simulink subsystem "Sustainer_Aerodynamics_old"  (R2023b)
settings: Solver=VariableStepAuto  StartTime=0.0  StopTime=10.0  RelTol=1e-3
undefined symbols (not defined in the file): ALPHA_axis3, ALT_axis1, CA_sustainer, CAQ_sustainer, CLL_sustainer, CLN_sustainer, CLP_sustainer, CLR_sustainer, CM_sustainer, CMAD_sustainer, CMQ_sustainer, CN_sustainer, CNAD_sustainer, CNP_sustainer, CNQ_sustainer, CNR_sustainer, CY_sustainer, CYP_sustainer, CYR_sustainer, F, Light, LREF, MIL, PHI_axis2, SREF, XCG_dry, XCP_sustainer
libraries: aerolibconvert2 x5, aerolibasang x2, simulink_extras x2, aerolibadyn x1, aerolibatmos2 x1, aerolibwind2 x1
settings Model: Creator=Andrew Radulovich  LastModifiedBy=thatf
settings ModelReferenceCC: EnableRefExpFcnMdlSchedulingChecks=on

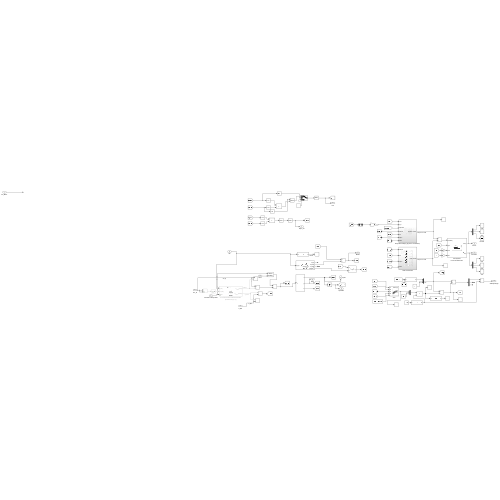
[thumbnail: Simulink's stored preview of the top-level diagram]
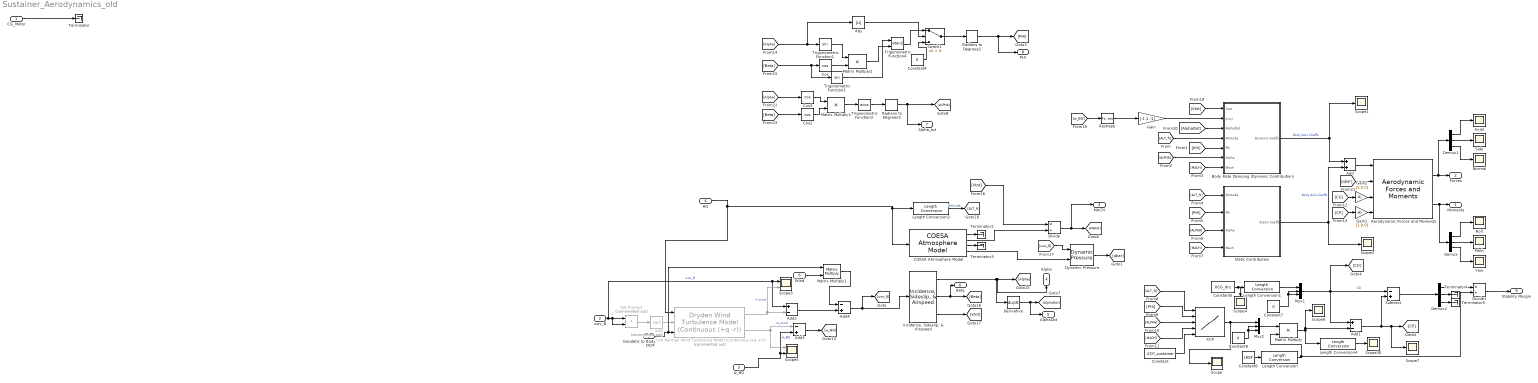
== system Sustainer_Aerodynamics_old ==
  CG_Motor : Inport
  uwv_B : Inport  Port=2
  w_BG : Inport  Port=3
  HG : Inport  Port=4
  Geodetic to Body DCM : Inport  Port=5
  Wind : Inport  Port=6
  Abs : Abs  SaturateOnIntegerOverflow=off
  Add : Sum
  Add1 : Sum  Inputs=+-
  Add2 : Sum  Inputs=+-
  Add3 : Sum  Inputs=-+
  Add4 : Sum  Inputs=-+
  "Aerodynamic Forces and Moments " : aerolibadyn/Aerodynamic Forces and Moments   inputAxes=Body  outputForceAxes=Body  outputMomentAxes=Body  S=SREF*0.0254*0.0254  b=LREF*0.0254  cbar=LREF*0.0254
  Axial : Scope
  "Body Rate Damping (Dynamic Contribution) " : Subsystem
  COESA Atmosphere Model : aerolibatmos2/COESA Atmosphere Model  units=Metric (MKS)  spec=1976 COESA-extended U.S. Standard Atmosphere  model=Profile  profile_var=High temperature  profile_percent=1%  profile_alt=5 km (16404 ft)  envelope_var=High temperature  envelope_percent=1%  action=None
  Constant : Constant  Value=XCP_sustainer  VectorParams1D=off
  Constant4 : Constant  Value=0
  Constant5 : Constant  Value=XCG_dry
  Constant6 : Constant  Value=LREF
  Constant7 : Constant  Value=0
  Constant8 : Constant  Value=0
  Cos : Trigonometry  Operator=cos
  Cos2 : Trigonometry  Operator=cos
  Cos3 : Trigonometry  Operator=cos
  Demux : Demux  Outputs=3
  Demux1 : Demux  Outputs=3
  Demux2 : Demux  Outputs=3
  Derivative : Derivative
  Divide : Product  Inputs=*/
  Divide1 : Product  Inputs=*/
  Dot Product : DotProduct  Commented=on  OutDataTypeStr=Inherit: Inherit via internal rule
  Dynamic Pressure : aerolibasang/Dynamic Pressure
  Gain : Gain  Gain=[-1,1,-1]
  Gain1 : Gain  Gain=[1,0,0]
  Gain2 : Gain  Gain=[1,0,0]
  "Incidence, Sideslip, & Airspeed" : aerolibasang/Incidence, Sideslip, & Airspeed
  Length Conversion : aerolibconvert2/Length Conversion  IU=in  OU=m
  Length Conversion1 : aerolibconvert2/Length Conversion  IU=in  OU=m
  Length Conversion2 : aerolibconvert2/Length Conversion  IU=m  OU=ft
  Length Conversion4 : aerolibconvert2/Length Conversion  IU=m  OU=in
  Matrix Multiply : Product
  Matrix Multiply1 : Product  Multiplication=Matrix(*)
  Matrix Multiply2 : Product
  Matrix Multiply3 : Product
  Mux1 : Mux  Inputs=3
  Mux2 : Mux  Inputs=3
  Normal : Scope
  Pitch : Scope
  Radians to Degrees2 : simulink_extras/Transformations/Radians to Degrees
  Radians to Degrees3 : simulink_extras/Transformations/Radians to Degrees
  Reshape : Reshape  OutputDimensionality=Row vector (2-D)
  Roll : Scope
  Scope{,1..2,4,6..7,30} (7 alike) : Scope
  Scope3 : Scope  NumInputPorts=2
  Scope5 : Scope  NumInputPorts=2
  Side : Scope
  Sqrt : Sqrt  Commented=on
  Static Contribution : Subsystem
  Subtract : Sum  Inputs=-+
  Switch1 : Switch  Criteria=u2 > Threshold  SaturateOnIntegerOverflow=off  InputSameDT=off
  Terminator{,2..5} (5 alike) : Terminator
  Trigonometric Function1 : Trigonometry
  Trigonometric Function2 : Trigonometry
  Trigonometric Function3 : Trigonometry  Operator=acos
  Trigonometric Function4 : Trigonometry  Operator=atan2
  Von Karman Wind Turbulence Model (Continuous (+q +r)) : aerolibwind2/Dryden Wind Turbulence Model  (Continuous (+q -r))  Commented=on  units=Metric (MKS)  spec=MIL-F-8785C  model=Continuous Von Karman (+q +r)  W20=15  Wdeg=0  TurbProb=10^-2 - Light  L_high=762  Wingspan=10  ts=0.1  Seed=[23341 23342 23343 23344]  T_on=on
  XCP : Lookup_n-D  NumberOfTableDimensions=4  BreakpointsForDimension1=ALT_axis1  BreakpointsForDimension2=PHI_axis2  BreakpointsForDimension3=ALPHA_axis3  BreakpointsForDimension4=MACH_axis4  TableSource=Input port  Table=reshape(repmat([4 5 6;16 19 20;10 18 23],1,2),[3,3,2])  InternalRulePriority=Speed  RndMeth=Simplest
      settings: InputPortMap=u0,u1,u2,u3,p221
  Yaw : Scope
  Moments : Outport
  Forces : Outport  Port=2
  MACH : Outport  Port=3
  Alpha : Outport  Port=4
  AlphaDot : Outport  Port=5
  Beta : Outport  Port=6
  Alpha_tot : Outport  Port=7
  PHI : Outport  Port=8
  Stability Margin : Outport  Port=9
  wires:
  CG_Motor/1 -> Terminator/1
  [ALPHA] -> XCP/3
  Abs/1 -> Switch1/2
  XCP/1 -> Scope/1, Mux2/1
  Divide/1 -> [MACH], MACH/1
  [Alpha] -> Cos3/1
  Trigonometric Function4/1 -> Switch1/1
  Cos3/1 -> Matrix Multiply3/1
  [uwv_B] -> Dynamic Pressure/1
  "Incidence, Sideslip, & Airspeed"/2 -> [Beta], Beta/1
  Trigonometric Function2/1 -> Trigonometric Function4/1
  Dynamic Pressure/1 -> [qbar]
  Gain/1 -> "Body Rate Damping (Dynamic Contribution) "/2(p,q,r)
  Length Conversion2/1 -> [ALT_ft]  "Altitude"
  COESA Atmosphere Model/3 -> Terminator3/1
  Static Contribution/1(Static Coeffs) -> Scope2/1, Add/2  "Body Axis Coeffs"
  Length Conversion/1 -> Matrix Multiply/2, Divide1/2
  Switch1/1 -> Radians to Degrees2/1
  [PHI] -> Static Contribution/2(Phi)
  [CP] -> Gain1/1
  Constant4/1 -> Switch1/3
  Gain1/1 -> "Aerodynamic Forces and Moments "/4
  Demux1/2 -> Side/1
  Constant6/1 -> Length Conversion/1
  [CG] -> Gain2/1
  Radians to Degrees2/1 -> [PHI], PHI/1
  Demux1/1 -> Axial/1
  [MACH] -> XCP/4
  Mux2/1 -> Matrix Multiply/1
  Add1/1 -> [CP], Scope7/1, Subtract/2
  "Aerodynamic Forces and Moments "/2 -> Demux/1, Moments/1
  Matrix Multiply/1 -> Length Conversion4/1, Add1/2, Scope6/1
  [MACH] -> Static Contribution/4(Mach)
  [PHI] -> XCP/2
  Gain2/1 -> "Aerodynamic Forces and Moments "/3
  "Incidence, Sideslip, & Airspeed"/1 -> Derivative/1, [Alpha], Alpha/1
  [AlphaDot] -> "Body Rate Damping (Dynamic Contribution) "/3(AlphaDot)
  Length Conversion1/1 -> Mux1/1
  Demux/3 -> Yaw/1
  Demux1/3 -> Normal/1
  [Vtot] -> "Body Rate Damping (Dynamic Contribution) "/1(Vtot)
  "Body Rate Damping (Dynamic Contribution) "/1("Dynamic Coeffs ") -> Add/1, Scope1/1  "Body Axis Coeffs"
  [ALT_ft] -> "Body Rate Damping (Dynamic Contribution) "/4(Altitude)
  Constant/1 -> XCP/5
  [Beta] -> Trigonometric Function2/1, Cos/1
  [qbar] -> "Aerodynamic Forces and Moments "/2
  Add/1 -> "Aerodynamic Forces and Moments "/1
  [ALT_ft] -> XCP/1
  Length Conversion4/1 -> Scope30/1
  Matrix Multiply3/1 -> Trigonometric Function3/1
  Cos/1 -> Matrix Multiply2/2
  Derivative/1 -> [AlphaDot], AlphaDot/1
  HG/1 -> Length Conversion2/1, COESA Atmosphere Model/1, Von Karman Wind Turbulence Model (Continuous (+q +r))/1
  Constant7/1 -> Mux1/2, Mux1/3
  Dot Product/1 -> Sqrt/1
  Cos2/1 -> Matrix Multiply3/2
  COESA Atmosphere Model/2 -> Divide/2
  [MACH] -> "Body Rate Damping (Dynamic Contribution) "/7(Mach)
  w_BG/1 -> Scope5/2, Add3/2  "w_BG"
  Trigonometric Function1/1 -> Matrix Multiply2/1
  Mux1/1 -> Add1/1, [CG], Subtract/1  "CG"
  Radians to Degrees3/1 -> [ALPHA], Alpha_tot/1
  Demux/1 -> Roll/1
  Trigonometric Function3/1 -> Radians to Degrees3/1
  Add2/1 -> Add4/2
  Matrix Multiply1/1 -> Add4/1
  Wind/1 -> Matrix Multiply1/2
  [PHI] -> "Body Rate Damping (Dynamic Contribution) "/5(Phi)
  "Incidence, Sideslip, & Airspeed"/3 -> [Vtot]
  COESA Atmosphere Model/4 -> Dynamic Pressure/2
  [ALPHA] -> "Body Rate Damping (Dynamic Contribution) "/6(Alpha)
  Add3/1 -> [w_BG]
  COESA Atmosphere Model/1 -> Terminator2/1
  Sqrt/1 -> Von Karman Wind Turbulence Model (Continuous (+q +r))/2
  Constant5/1 -> Length Conversion1/1, Scope4/1
  [Beta] -> Cos2/1
  Von Karman Wind Turbulence Model (Continuous (+q +r))/2 -> Scope5/1, Add3/1  "w_wind"
  [Vtot] -> Divide/1
  [ALPHA] -> Static Contribution/3(Alpha)
  Add4/1 -> [uwv_B], "Incidence, Sideslip, & Airspeed"/1
  Reshape/1 -> Gain/1
  Matrix Multiply2/1 -> Trigonometric Function4/2
  Geodetic to Body DCM/1 -> Von Karman Wind Turbulence Model (Continuous (+q +r))/3, Matrix Multiply1/1
  Demux/2 -> Pitch/1
  [w_BG] -> Reshape/1
  uwv_B/1 -> Dot Product/1, Dot Product/2, Scope3/1, Add2/1  "uwv_B"
  [Alpha] -> Trigonometric Function1/1, Abs/1
  [ALT_ft] -> Static Contribution/1(Altitude)
  Constant8/1 -> Mux2/2, Mux2/3
  "Aerodynamic Forces and Moments "/1 -> Forces/1, Demux1/1
  Von Karman Wind Turbulence Model (Continuous (+q +r))/1 -> Scope3/2, Add2/2  "V wind"
  Subtract/1 -> Demux2/1
  Demux2/1 -> Divide1/1
  Demux2/2 -> Terminator4/1
  Demux2/3 -> Terminator5/1
  Divide1/1 -> Stability Margin/1

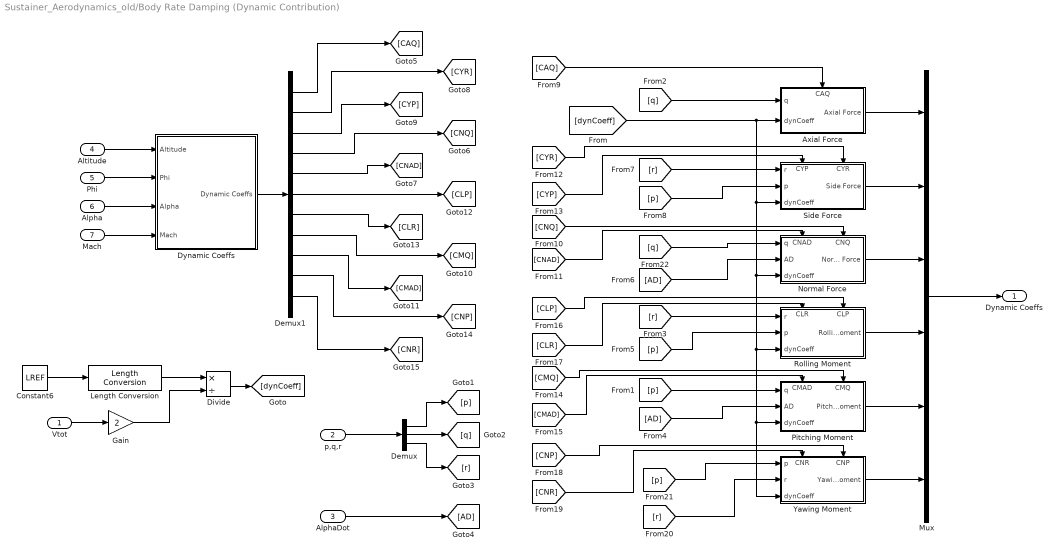
== system Sustainer_Aerodynamics_old/Body Rate Damping (Dynamic Contribution)  ==
  Vtot : Inport
  p,q,r : Inport  Port=2
  AlphaDot : Inport  Port=3
  Altitude : Inport  Port=4
  Phi : Inport  Port=5
  Alpha : Inport  Port=6
  Mach : Inport  Port=7
  Axial Force : Subsystem
      settings: PortSchema="{\"entries\":[{\"content\":{\"sides\":[{\"content\":{\"connectorIds\":[\"In1\",\"In2\"]},\"type\":\"ConnectorPlacement.EquallySpacedRectSide\",\"uuid\":\"567ace9e-aa72-447b-a995-1912c2144b72\"},{\"content\":{\"connectorIds\":[\"Out1\"],\"side\":\"RIGHT\"},\"type\":\"ConnectorPlacement.EquallySpacedRectSide\",\"uuid\":\"f61a370b-a555-422d-b0aa-b7ff6aed3edf\"},{\"content\":{\"connectorIds\":[\"In3\"],\"side\":\"TOP\"},\"type\":\"ConnectorPlacement.EquallySpacedRectSide\",\"uuid\":\"bbb221a2-e351-4e94-b4cf-9d8a77c477bc\"}]},\"type\":\"ConnectorPlacement.EquallySpacedConnector\",\"uuid\":\"32afc2d8-df0e-48c6-a674-90055023081f\"}],\"packageUris\":[\"http://schema.mathworks.com/mf0/Connector/R2020b\"],\"version\":\"1.0\"}"
  Constant6 : Constant  Value=LREF
  Demux : Demux  Outputs=3
  Demux1 : Demux  Outputs=11
  Divide : Product  Inputs=*/
  Dynamic Coeffs : Subsystem
  Gain : Gain  Gain=2
  Length Conversion : aerolibconvert2/Length Conversion  IU=in  OU=m
  Mux : Mux  Inputs=6
  Normal Force : Subsystem
      settings: PortSchema="{\"entries\":[{\"content\":{\"sides\":[{\"content\":{\"connectorIds\":[\"In1\",\"In2\",\"In3\"]},\"type\":\"ConnectorPlacement.EquallySpacedRectSide\",\"uuid\":\"36c1ca9e-f728-46fa-a5e1-3a4eef93369b\"},{\"content\":{\"connectorIds\":[\"Out1\"],\"side\":\"RIGHT\"},\"type\":\"ConnectorPlacement.EquallySpacedRectSide\",\"uuid\":\"48421245-83fe-4d4e-9595-34bafe35022f\"},{\"content\":{\"connectorIds\":[\"In4\",\"In5\"],\"side\":\"TOP\"},\"type\":\"ConnectorPlacement.EquallySpacedRectSide\",\"uuid\":\"de332918-1e12-41a2-8ccc-a9221aaa9415\"}]},\"type\":\"ConnectorPlacement.EquallySpacedConnector\",\"uuid\":\"0485d59f-61a8-483f-be32-e9ca6bf2e6bf\"}],\"packageUris\":[\"http://schema.mathworks.com/mf0/Connector/R2020b\"],\"version\":\"1.0\"}"
  Pitching Moment : Subsystem
      settings: PortSchema="{\"entries\":[{\"content\":{\"sides\":[{\"content\":{\"connectorIds\":[\"In1\",\"In2\",\"In3\"]},\"type\":\"ConnectorPlacement.EquallySpacedRectSide\",\"uuid\":\"36c1ca9e-f728-46fa-a5e1-3a4eef93369b\"},{\"content\":{\"connectorIds\":[\"Out1\"],\"side\":\"RIGHT\"},\"type\":\"ConnectorPlacement.EquallySpacedRectSide\",\"uuid\":\"48421245-83fe-4d4e-9595-34bafe35022f\"},{\"content\":{\"connectorIds\":[\"In4\",\"In5\"],\"side\":\"TOP\"},\"type\":\"ConnectorPlacement.EquallySpacedRectSide\",\"uuid\":\"de332918-1e12-41a2-8ccc-a9221aaa9415\"}]},\"type\":\"ConnectorPlacement.EquallySpacedConnector\",\"uuid\":\"0485d59f-61a8-483f-be32-e9ca6bf2e6bf\"}],\"packageUris\":[\"http://schema.mathworks.com/mf0/Connector/R2020b\"],\"version\":\"1.0\"}"
  Rolling Moment : Subsystem
      settings: PortSchema="{\"entries\":[{\"content\":{\"sides\":[{\"content\":{\"connectorIds\":[\"In1\",\"In2\",\"In3\"]},\"type\":\"ConnectorPlacement.EquallySpacedRectSide\",\"uuid\":\"36c1ca9e-f728-46fa-a5e1-3a4eef93369b\"},{\"content\":{\"connectorIds\":[\"Out1\"],\"side\":\"RIGHT\"},\"type\":\"ConnectorPlacement.EquallySpacedRectSide\",\"uuid\":\"48421245-83fe-4d4e-9595-34bafe35022f\"},{\"content\":{\"connectorIds\":[\"In4\",\"In5\"],\"side\":\"TOP\"},\"type\":\"ConnectorPlacement.EquallySpacedRectSide\",\"uuid\":\"de332918-1e12-41a2-8ccc-a9221aaa9415\"}]},\"type\":\"ConnectorPlacement.EquallySpacedConnector\",\"uuid\":\"0485d59f-61a8-483f-be32-e9ca6bf2e6bf\"}],\"packageUris\":[\"http://schema.mathworks.com/mf0/Connector/R2020b\"],\"version\":\"1.0\"}"
  Side Force : Subsystem
      settings: PortSchema="{\"entries\":[{\"content\":{\"sides\":[{\"content\":{\"connectorIds\":[\"In1\",\"In2\",\"In3\"]},\"type\":\"ConnectorPlacement.EquallySpacedRectSide\",\"uuid\":\"36c1ca9e-f728-46fa-a5e1-3a4eef93369b\"},{\"content\":{\"connectorIds\":[\"Out1\"],\"side\":\"RIGHT\"},\"type\":\"ConnectorPlacement.EquallySpacedRectSide\",\"uuid\":\"48421245-83fe-4d4e-9595-34bafe35022f\"},{\"content\":{\"connectorIds\":[\"In4\",\"In5\"],\"side\":\"TOP\"},\"type\":\"ConnectorPlacement.EquallySpacedRectSide\",\"uuid\":\"de332918-1e12-41a2-8ccc-a9221aaa9415\"}]},\"type\":\"ConnectorPlacement.EquallySpacedConnector\",\"uuid\":\"0485d59f-61a8-483f-be32-e9ca6bf2e6bf\"}],\"packageUris\":[\"http://schema.mathworks.com/mf0/Connector/R2020b\"],\"version\":\"1.0\"}"
  Yawing Moment : Subsystem
      settings: PortSchema="{\"entries\":[{\"content\":{\"sides\":[{\"content\":{\"connectorIds\":[\"In1\",\"In2\",\"In3\"]},\"type\":\"ConnectorPlacement.EquallySpacedRectSide\",\"uuid\":\"36c1ca9e-f728-46fa-a5e1-3a4eef93369b\"},{\"content\":{\"connectorIds\":[\"Out1\"],\"side\":\"RIGHT\"},\"type\":\"ConnectorPlacement.EquallySpacedRectSide\",\"uuid\":\"48421245-83fe-4d4e-9595-34bafe35022f\"},{\"content\":{\"connectorIds\":[\"In4\",\"In5\"],\"side\":\"TOP\"},\"type\":\"ConnectorPlacement.EquallySpacedRectSide\",\"uuid\":\"de332918-1e12-41a2-8ccc-a9221aaa9415\"}]},\"type\":\"ConnectorPlacement.EquallySpacedConnector\",\"uuid\":\"0485d59f-61a8-483f-be32-e9ca6bf2e6bf\"}],\"packageUris\":[\"http://schema.mathworks.com/mf0/Connector/R2020b\"],\"version\":\"1.0\"}"
  "Dynamic Coeffs " : Outport
  wires:
  Yawing Moment/1(Yawing Moment) -> Mux/6
  Pitching Moment/1(Pitching Moment) -> Mux/5
  Rolling Moment/1(Rolling Moment) -> Mux/4
  Normal Force/1(Normal Force) -> Mux/3
  Side Force/1(Side Force) -> Mux/2
  Axial Force/1(Axial Force) -> Mux/1
  [q] -> Normal Force/1(q)
  [r] -> Yawing Moment/2(r)
  [p] -> Yawing Moment/1(p)
  [r] -> Rolling Moment/1(r)
  [CLR] -> Rolling Moment/4(CLR)
  [CLP] -> Rolling Moment/5(CLP)
  [p] -> Rolling Moment/2(p)
  [CMAD] -> Pitching Moment/4(CMAD)
  [CMQ] -> Pitching Moment/5(CMQ)
  [p] -> Pitching Moment/1(q)
  [AD] -> Pitching Moment/2(AD)
  [CYR] -> Side Force/5(CYR)
  [r] -> Side Force/1(r)
  [CYP] -> Side Force/4(CYP)
  [p] -> Side Force/2(p)
  [CNAD] -> Normal Force/4(CNAD)
  [CNQ] -> Normal Force/5(CNQ)
  [AD] -> Normal Force/2(AD)
  Demux1/11 -> [CNR]
  Demux1/10 -> [CNP]
  Demux1/9 -> [CMAD]
  Demux1/8 -> [CMQ]
  Demux1/7 -> [CLR]
  Demux1/6 -> [CLP]
  Demux1/5 -> [CNAD]
  Demux1/4 -> [CNQ]
  Demux1/3 -> [CYP]
  Demux1/2 -> [CYR]
  [CNR] -> Yawing Moment/4(CNR)
  [CNP] -> Yawing Moment/5(CNP)
  [CAQ] -> Axial Force/3(CAQ)
  Demux1/1 -> [CAQ]
  Dynamic Coeffs/1(Dynamic Coeffs) -> Demux1/1
  Mach/1 -> Dynamic Coeffs/4(Mach)
  Alpha/1 -> Dynamic Coeffs/3(Alpha)
  Phi/1 -> Dynamic Coeffs/2(Phi)
  Altitude/1 -> Dynamic Coeffs/1(Altitude)
  Mux/1 -> "Dynamic Coeffs "/1
  [dynCoeff] -> Axial Force/2(dynCoeff), Normal Force/3(dynCoeff), Rolling Moment/3(dynCoeff), Yawing Moment/3(dynCoeff), Pitching Moment/3(dynCoeff), Side Force/3(dynCoeff)
  [q] -> Axial Force/1(q)
  AlphaDot/1 -> [AD]
  Vtot/1 -> Gain/1
  p,q,r/1 -> Demux/1
  Demux/1 -> [p]
  Constant6/1 -> Length Conversion/1
  Divide/1 -> [dynCoeff]
  Demux/2 -> [q]
  Demux/3 -> [r]
  Length Conversion/1 -> Divide/1
  Gain/1 -> Divide/2

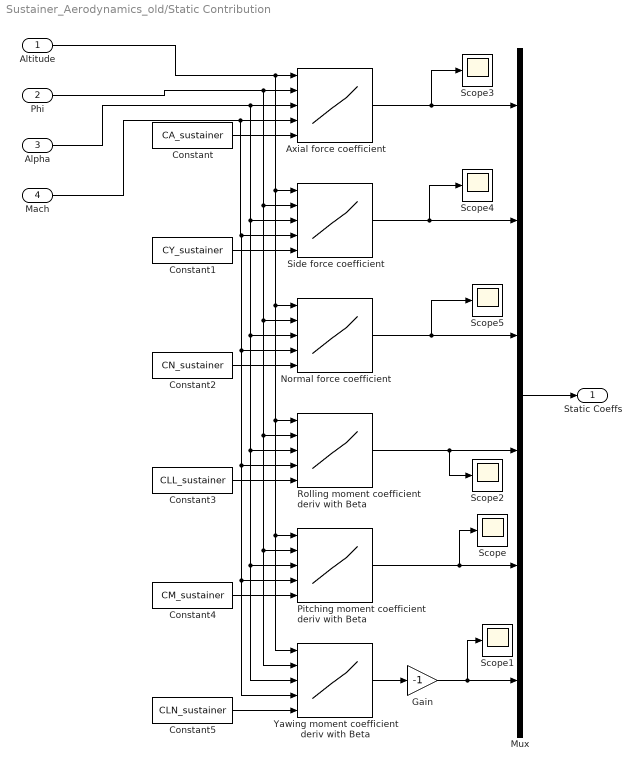
== system Sustainer_Aerodynamics_old/Static Contribution ==
  Altitude : Inport
  Phi : Inport  Port=2
  Alpha : Inport  Port=3
  Mach : Inport  Port=4
  Axial force coefficient : Lookup_n-D  NumberOfTableDimensions=4  BreakpointsForDimension1=ALT_axis1  BreakpointsForDimension2=PHI_axis2  BreakpointsForDimension3=ALPHA_axis3  BreakpointsForDimension4=MACH_axis4  TableSource=Input port  Table=reshape(repmat([4 5 6;16 19 20;10 18 23],1,2),[3,3,2])  DiagnosticForOutOfRangeInput=Warning  InternalRulePriority=Speed  RndMeth=Simplest
      settings: InputPortMap=u0,u1,u2,u3,p221
  Constant : Constant  Value=CA_sustainer  VectorParams1D=off
  Constant1 : Constant  Value=CY_sustainer  VectorParams1D=off
  Constant2 : Constant  Value=CN_sustainer  VectorParams1D=off
  Constant3 : Constant  Value=CLL_sustainer  VectorParams1D=off
  Constant4 : Constant  Value=CM_sustainer  VectorParams1D=off
  Constant5 : Constant  Value=CLN_sustainer  VectorParams1D=off
  Gain : Gain  Gain=-1
  Mux : Mux  Inputs=6
  Normal force coefficient : Lookup_n-D  NumberOfTableDimensions=4  BreakpointsForDimension1=ALT_axis1  BreakpointsForDimension2=PHI_axis2  BreakpointsForDimension3=ALPHA_axis3  BreakpointsForDimension4=MACH_axis4  TableSource=Input port  Table=reshape(repmat([4 5 6;16 19 20;10 18 23],1,2),[3,3,2])  InternalRulePriority=Speed  RndMeth=Simplest
      settings: InputPortMap=u0,u1,u2,u3,p221
  Pitching moment coefficient deriv with Beta : Lookup_n-D  NumberOfTableDimensions=4  BreakpointsForDimension1=ALT_axis1  BreakpointsForDimension2=PHI_axis2  BreakpointsForDimension3=ALPHA_axis3  BreakpointsForDimension4=MACH_axis4  TableSource=Input port  Table=reshape(repmat([4 5 6;16 19 20;10 18 23],1,2),[3,3,2])  InternalRulePriority=Speed  RndMeth=Simplest
      settings: InputPortMap=u0,u1,u2,u3,p221
  Rolling moment coefficient deriv with Beta : Lookup_n-D  NumberOfTableDimensions=4  BreakpointsForDimension1=ALT_axis1  BreakpointsForDimension2=PHI_axis2  BreakpointsForDimension3=ALPHA_axis3  BreakpointsForDimension4=MACH_axis4  TableSource=Input port  Table=reshape(repmat([4 5 6;16 19 20;10 18 23],1,2),[3,3,2])  InterpMethod=Linear Lagrange  InternalRulePriority=Speed  RndMeth=Simplest
      settings: InputPortMap=u0,u1,u2,u3,p221
  Scope{,1..5} (6 alike) : Scope
  Side force coefficient : Lookup_n-D  NumberOfTableDimensions=4  BreakpointsForDimension1=ALT_axis1  BreakpointsForDimension2=PHI_axis2  BreakpointsForDimension3=ALPHA_axis3  BreakpointsForDimension4=MACH_axis4  TableSource=Input port  Table=reshape(repmat([4 5 6;16 19 20;10 18 23],1,2),[3,3,2])  InternalRulePriority=Speed  RndMeth=Simplest
      settings: InputPortMap=u0,u1,u2,u3,p221
  Yawing moment coefficient deriv with Beta : Lookup_n-D  NumberOfTableDimensions=4  BreakpointsForDimension1=ALT_axis1  BreakpointsForDimension2=PHI_axis2  BreakpointsForDimension3=ALPHA_axis3  BreakpointsForDimension4=MACH_axis4  TableSource=Input port  Table=reshape(repmat([4 5 6;16 19 20;10 18 23],1,2),[3,3,2])  InternalRulePriority=Speed  RndMeth=Simplest
      settings: InputPortMap=u0,u1,u2,u3,p221
  Static Coeffs : Outport
  wires:
  Alpha/1 -> Rolling moment coefficient deriv with Beta/3, Pitching moment coefficient deriv with Beta/3, Yawing moment coefficient deriv with Beta/3, Normal force coefficient/3, Side force coefficient/3, Axial force coefficient/3
  Mach/1 -> Axial force coefficient/4, Side force coefficient/4, Normal force coefficient/4, Rolling moment coefficient deriv with Beta/4, Pitching moment coefficient deriv with Beta/4, Yawing moment coefficient deriv with Beta/4
  Phi/1 -> Normal force coefficient/2, Rolling moment coefficient deriv with Beta/2, Pitching moment coefficient deriv with Beta/2, Yawing moment coefficient deriv with Beta/2, Side force coefficient/2, Axial force coefficient/2
  Altitude/1 -> Axial force coefficient/1, Side force coefficient/1, Rolling moment coefficient deriv with Beta/1, Pitching moment coefficient deriv with Beta/1, Yawing moment coefficient deriv with Beta/1, Normal force coefficient/1
  Pitching moment coefficient deriv with Beta/1 -> Mux/5, Scope/1
  Rolling moment coefficient deriv with Beta/1 -> Mux/4, Scope2/1
  Side force coefficient/1 -> Mux/2, Scope4/1
  Constant/1 -> Axial force coefficient/5
  Normal force coefficient/1 -> Mux/3, Scope5/1
  Constant5/1 -> Yawing moment coefficient deriv with Beta/5
  Mux/1 -> Static Coeffs/1
  Axial force coefficient/1 -> Mux/1, Scope3/1
  Constant4/1 -> Pitching moment coefficient deriv with Beta/5
  Constant3/1 -> Rolling moment coefficient deriv with Beta/5
  Constant2/1 -> Normal force coefficient/5
  Constant1/1 -> Side force coefficient/5
  Yawing moment coefficient deriv with Beta/1 -> Gain/1
  Gain/1 -> Scope1/1, Mux/6

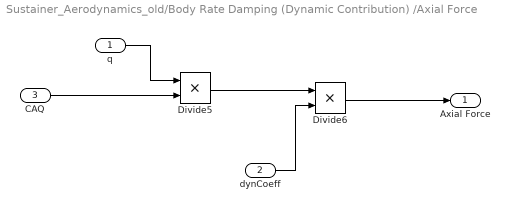
== system Sustainer_Aerodynamics_old/Body Rate Damping (Dynamic Contribution) /Axial Force ==
  q : Inport
  dynCoeff : Inport  Port=2
  CAQ : Inport  Port=3
  Divide5 : Product  Inputs=**
  Divide6 : Product  Inputs=**
  Axial Force : Outport
  wires:
  CAQ/1 -> Divide5/2
  Divide6/1 -> Axial Force/1
  q/1 -> Divide5/1
  Divide5/1 -> Divide6/1
  dynCoeff/1 -> Divide6/2

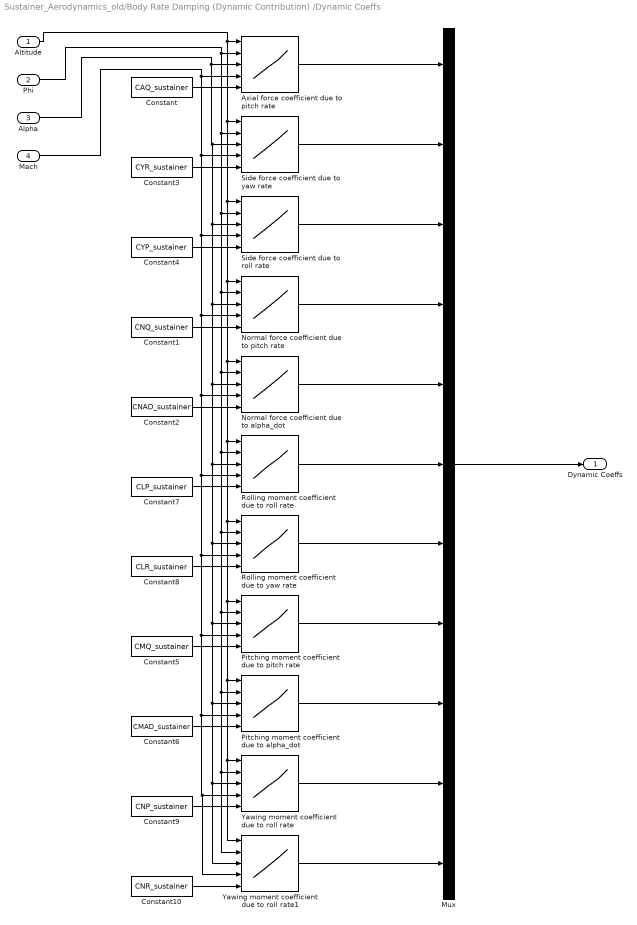
== system Sustainer_Aerodynamics_old/Body Rate Damping (Dynamic Contribution) /Dynamic Coeffs ==
  Altitude : Inport
  Phi : Inport  Port=2
  Alpha : Inport  Port=3
  Mach : Inport  Port=4
  Axial force coefficient due to pitch rate : Lookup_n-D  NumberOfTableDimensions=4  BreakpointsForDimension1=ALT_axis1  BreakpointsForDimension2=PHI_axis2  BreakpointsForDimension3=ALPHA_axis3  BreakpointsForDimension4=MACH_axis4  TableSource=Input port  Table=reshape(repmat([4 5 6;16 19 20;10 18 23],1,2),[3,3,2])  InternalRulePriority=Speed  RndMeth=Simplest
      settings: InputPortMap=u0,u1,u2,u3,p221
  Constant : Constant  Value=CAQ_sustainer  VectorParams1D=off
  Constant1 : Constant  Value=CNQ_sustainer  VectorParams1D=off
  Constant10 : Constant  Value=CNR_sustainer  VectorParams1D=off
  Constant2 : Constant  Value=CNAD_sustainer  VectorParams1D=off
  Constant3 : Constant  Value=CYR_sustainer  VectorParams1D=off
  Constant4 : Constant  Value=CYP_sustainer  VectorParams1D=off
  Constant5 : Constant  Value=CMQ_sustainer  VectorParams1D=off
  Constant6 : Constant  Value=CMAD_sustainer  VectorParams1D=off
  Constant7 : Constant  Value=CLP_sustainer  VectorParams1D=off
  Constant8 : Constant  Value=CLR_sustainer  VectorParams1D=off
  Constant9 : Constant  Value=CNP_sustainer  VectorParams1D=off
  Mux : Mux  Inputs=11
  Normal force coefficient due to alpha_dot : Lookup_n-D  NumberOfTableDimensions=4  BreakpointsForDimension1=ALT_axis1  BreakpointsForDimension2=PHI_axis2  BreakpointsForDimension3=ALPHA_axis3  BreakpointsForDimension4=MACH_axis4  TableSource=Input port  Table=reshape(repmat([4 5 6;16 19 20;10 18 23],1,2),[3,3,2])  InternalRulePriority=Speed  RndMeth=Simplest
      settings: InputPortMap=u0,u1,u2,u3,p221
  Normal force coefficient due to pitch rate : Lookup_n-D  NumberOfTableDimensions=4  BreakpointsForDimension1=ALT_axis1  BreakpointsForDimension2=PHI_axis2  BreakpointsForDimension3=ALPHA_axis3  BreakpointsForDimension4=MACH_axis4  TableSource=Input port  Table=reshape(repmat([4 5 6;16 19 20;10 18 23],1,2),[3,3,2])  InternalRulePriority=Speed  RndMeth=Simplest
      settings: InputPortMap=u0,u1,u2,u3,p221
  Pitching moment coefficient due to alpha_dot : Lookup_n-D  NumberOfTableDimensions=4  BreakpointsForDimension1=ALT_axis1  BreakpointsForDimension2=PHI_axis2  BreakpointsForDimension3=ALPHA_axis3  BreakpointsForDimension4=MACH_axis4  TableSource=Input port  Table=reshape(repmat([4 5 6;16 19 20;10 18 23],1,2),[3,3,2])  InternalRulePriority=Speed  RndMeth=Simplest
      settings: InputPortMap=u0,u1,u2,u3,p221
  Pitching moment coefficient due to pitch rate : Lookup_n-D  NumberOfTableDimensions=4  BreakpointsForDimension1=ALT_axis1  BreakpointsForDimension2=PHI_axis2  BreakpointsForDimension3=ALPHA_axis3  BreakpointsForDimension4=MACH_axis4  TableSource=Input port  Table=reshape(repmat([4 5 6;16 19 20;10 18 23],1,2),[3,3,2])  InternalRulePriority=Speed  RndMeth=Simplest
      settings: InputPortMap=u0,u1,u2,u3,p221
  Rolling moment coefficient due to roll rate : Lookup_n-D  NumberOfTableDimensions=4  BreakpointsForDimension1=ALT_axis1  BreakpointsForDimension2=PHI_axis2  BreakpointsForDimension3=ALPHA_axis3  BreakpointsForDimension4=MACH_axis4  TableSource=Input port  Table=reshape(repmat([4 5 6;16 19 20;10 18 23],1,2),[3,3,2])  InterpMethod=Linear Lagrange  InternalRulePriority=Speed  RndMeth=Simplest
      settings: InputPortMap=u0,u1,u2,u3,p221
  Rolling moment coefficient due to yaw rate : Lookup_n-D  NumberOfTableDimensions=4  BreakpointsForDimension1=ALT_axis1  BreakpointsForDimension2=PHI_axis2  BreakpointsForDimension3=ALPHA_axis3  BreakpointsForDimension4=MACH_axis4  TableSource=Input port  Table=reshape(repmat([4 5 6;16 19 20;10 18 23],1,2),[3,3,2])  InterpMethod=Linear Lagrange  InternalRulePriority=Speed  RndMeth=Simplest
      settings: InputPortMap=u0,u1,u2,u3,p221
  Side force coefficient due to roll rate : Lookup_n-D  NumberOfTableDimensions=4  BreakpointsForDimension1=ALT_axis1  BreakpointsForDimension2=PHI_axis2  BreakpointsForDimension3=ALPHA_axis3  BreakpointsForDimension4=MACH_axis4  TableSource=Input port  Table=reshape(repmat([4 5 6;16 19 20;10 18 23],1,2),[3,3,2])  InternalRulePriority=Speed  RndMeth=Simplest
      settings: InputPortMap=u0,u1,u2,u3,p221
  Side force coefficient due to yaw rate : Lookup_n-D  NumberOfTableDimensions=4  BreakpointsForDimension1=ALT_axis1  BreakpointsForDimension2=PHI_axis2  BreakpointsForDimension3=ALPHA_axis3  BreakpointsForDimension4=MACH_axis4  TableSource=Input port  Table=reshape(repmat([4 5 6;16 19 20;10 18 23],1,2),[3,3,2])  InternalRulePriority=Speed  RndMeth=Simplest
      settings: InputPortMap=u0,u1,u2,u3,p221
  Yawing moment coefficient due to roll rate : Lookup_n-D  NumberOfTableDimensions=4  BreakpointsForDimension1=ALT_axis1  BreakpointsForDimension2=PHI_axis2  BreakpointsForDimension3=ALPHA_axis3  BreakpointsForDimension4=MACH_axis4  TableSource=Input port  Table=reshape(repmat([4 5 6;16 19 20;10 18 23],1,2),[3,3,2])  InternalRulePriority=Speed  RndMeth=Simplest
      settings: InputPortMap=u0,u1,u2,u3,p221
  Yawing moment coefficient due to roll rate1 : Lookup_n-D  NumberOfTableDimensions=4  BreakpointsForDimension1=ALT_axis1  BreakpointsForDimension2=PHI_axis2  BreakpointsForDimension3=ALPHA_axis3  BreakpointsForDimension4=MACH_axis4  TableSource=Input port  Table=reshape(repmat([4 5 6;16 19 20;10 18 23],1,2),[3,3,2])  InternalRulePriority=Speed  RndMeth=Simplest
      settings: InputPortMap=u0,u1,u2,u3,p221
  Dynamic Coeffs : Outport
  wires:
  Yawing moment coefficient due to roll rate1/1 -> Mux/11
  Yawing moment coefficient due to roll rate/1 -> Mux/10
  Pitching moment coefficient due to alpha_dot/1 -> Mux/9
  Pitching moment coefficient due to pitch rate/1 -> Mux/8
  Rolling moment coefficient due to yaw rate/1 -> Mux/7
  Constant10/1 -> Yawing moment coefficient due to roll rate1/5
  Constant9/1 -> Yawing moment coefficient due to roll rate/5
  Constant6/1 -> Pitching moment coefficient due to alpha_dot/5
  Constant5/1 -> Pitching moment coefficient due to pitch rate/5
  Constant8/1 -> Rolling moment coefficient due to yaw rate/5
  Altitude/1 -> Axial force coefficient due to pitch rate/1, Side force coefficient due to yaw rate/1, Side force coefficient due to roll rate/1, Normal force coefficient due to pitch rate/1, Normal force coefficient due to alpha_dot/1, Rolling moment coefficient due to roll rate/1, Rolling moment coefficient due to yaw rate/1, Pitching moment coefficient due to pitch rate/1, Pitching moment coefficient due to alpha_dot/1, Yawing moment coefficient due to roll rate/1, Yawing moment coefficient due to roll rate1/1
  Constant3/1 -> Side force coefficient due to yaw rate/5
  Phi/1 -> Axial force coefficient due to pitch rate/2, Side force coefficient due to yaw rate/2, Side force coefficient due to roll rate/2, Normal force coefficient due to pitch rate/2, Normal force coefficient due to alpha_dot/2, Rolling moment coefficient due to roll rate/2, Rolling moment coefficient due to yaw rate/2, Yawing moment coefficient due to roll rate1/2, Yawing moment coefficient due to roll rate/2, Pitching moment coefficient due to alpha_dot/2, Pitching moment coefficient due to pitch rate/2
  Constant/1 -> Axial force coefficient due to pitch rate/5
  Axial force coefficient due to pitch rate/1 -> Mux/1
  Side force coefficient due to roll rate/1 -> Mux/3
  Constant1/1 -> Normal force coefficient due to pitch rate/5
  Rolling moment coefficient due to roll rate/1 -> Mux/6
  Constant7/1 -> Rolling moment coefficient due to roll rate/5
  Normal force coefficient due to alpha_dot/1 -> Mux/5
  Side force coefficient due to yaw rate/1 -> Mux/2
  Constant4/1 -> Side force coefficient due to roll rate/5
  Constant2/1 -> Normal force coefficient due to alpha_dot/5
  Mux/1 -> Dynamic Coeffs/1
  Normal force coefficient due to pitch rate/1 -> Mux/4
  Alpha/1 -> Axial force coefficient due to pitch rate/3, Side force coefficient due to yaw rate/3, Side force coefficient due to roll rate/3, Normal force coefficient due to pitch rate/3, Normal force coefficient due to alpha_dot/3, Rolling moment coefficient due to roll rate/3, Rolling moment coefficient due to yaw rate/3, Yawing moment coefficient due to roll rate/3, Yawing moment coefficient due to roll rate1/3, Pitching moment coefficient due to alpha_dot/3, Pitching moment coefficient due to pitch rate/3
  Mach/1 -> Axial force coefficient due to pitch rate/4, Side force coefficient due to yaw rate/4, Side force coefficient due to roll rate/4, Normal force coefficient due to pitch rate/4, Normal force coefficient due to alpha_dot/4, Rolling moment coefficient due to roll rate/4, Pitching moment coefficient due to pitch rate/4, Pitching moment coefficient due to alpha_dot/4, Yawing moment coefficient due to roll rate/4, Yawing moment coefficient due to roll rate1/4, Rolling moment coefficient due to yaw rate/4

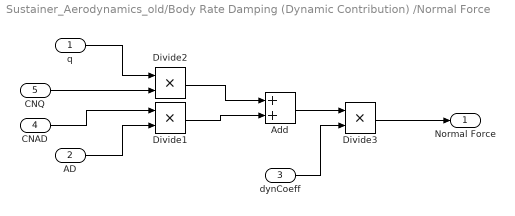
== system Sustainer_Aerodynamics_old/Body Rate Damping (Dynamic Contribution) /Normal Force ==
  q : Inport
  AD : Inport  Port=2
  dynCoeff : Inport  Port=3
  CNAD : Inport  Port=4
  CNQ : Inport  Port=5
  Add : Sum
  Divide1 : Product  Inputs=**
  Divide2 : Product  Inputs=**
  Divide3 : Product  Inputs=**
  Normal Force : Outport
  wires:
  CNAD/1 -> Divide1/1
  CNQ/1 -> Divide2/2
  q/1 -> Divide2/1
  dynCoeff/1 -> Divide3/2
  Divide1/1 -> Add/2
  AD/1 -> Divide1/2
  Add/1 -> Divide3/1
  Divide3/1 -> Normal Force/1
  Divide2/1 -> Add/1

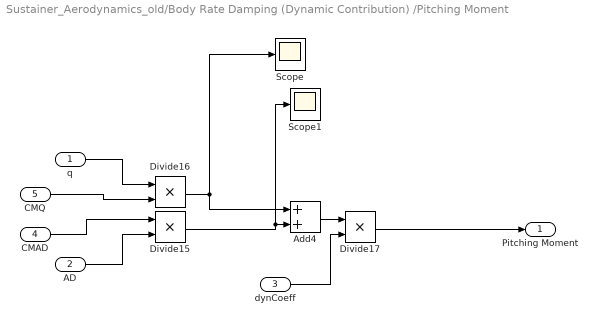
== system Sustainer_Aerodynamics_old/Body Rate Damping (Dynamic Contribution) /Pitching Moment ==
  q : Inport
  AD : Inport  Port=2
  dynCoeff : Inport  Port=3
  CMAD : Inport  Port=4
  CMQ : Inport  Port=5
  Add4 : Sum
  Divide15 : Product  Inputs=**
  Divide16 : Product  Inputs=**
  Divide17 : Product  Inputs=**
  Scope : Scope
  Scope1 : Scope
  Pitching Moment : Outport
  wires:
  CMAD/1 -> Divide15/1
  CMQ/1 -> Divide16/2
  Divide17/1 -> Pitching Moment/1
  dynCoeff/1 -> Divide17/2
  Divide15/1 -> Add4/2, Scope1/1
  Divide16/1 -> Add4/1, Scope/1
  AD/1 -> Divide15/2
  q/1 -> Divide16/1
  Add4/1 -> Divide17/1

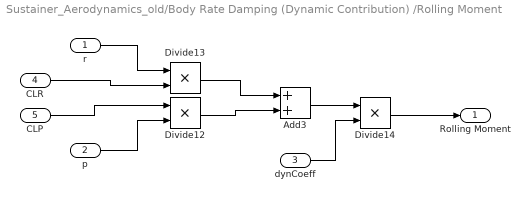
== system Sustainer_Aerodynamics_old/Body Rate Damping (Dynamic Contribution) /Rolling Moment ==
  r : Inport
  p : Inport  Port=2
  dynCoeff : Inport  Port=3
  CLR : Inport  Port=4
  CLP : Inport  Port=5
  Add3 : Sum
  Divide12 : Product  Inputs=**
  Divide13 : Product  Inputs=**
  Divide14 : Product  Inputs=**
  Rolling Moment : Outport
  wires:
  CLR/1 -> Divide13/2
  CLP/1 -> Divide12/1
  Divide14/1 -> Rolling Moment/1
  Add3/1 -> Divide14/1
  r/1 -> Divide13/1
  dynCoeff/1 -> Divide14/2
  Divide13/1 -> Add3/1
  Divide12/1 -> Add3/2
  p/1 -> Divide12/2

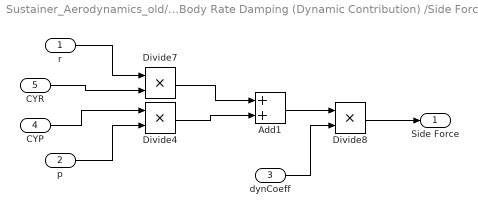
== system Sustainer_Aerodynamics_old/Body Rate Damping (Dynamic Contribution) /Side Force ==
  r : Inport
  p : Inport  Port=2
  dynCoeff : Inport  Port=3
  CYP : Inport  Port=4
  CYR : Inport  Port=5
  Add1 : Sum
  Divide4 : Product  Inputs=**
  Divide7 : Product  Inputs=**
  Divide8 : Product  Inputs=**
  Side Force : Outport
  wires:
  CYP/1 -> Divide4/1
  CYR/1 -> Divide7/2
  r/1 -> Divide7/1
  p/1 -> Divide4/2
  dynCoeff/1 -> Divide8/2
  Divide7/1 -> Add1/1
  Divide8/1 -> Side Force/1
  Add1/1 -> Divide8/1
  Divide4/1 -> Add1/2

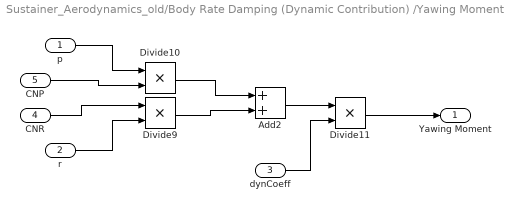
== system Sustainer_Aerodynamics_old/Body Rate Damping (Dynamic Contribution) /Yawing Moment ==
  p : Inport
  r : Inport  Port=2
  dynCoeff : Inport  Port=3
  CNR : Inport  Port=4
  CNP : Inport  Port=5
  Add2 : Sum
  Divide10 : Product  Inputs=**
  Divide11 : Product  Inputs=**
  Divide9 : Product  Inputs=**
  Yawing Moment : Outport
  wires:
  CNR/1 -> Divide9/1
  CNP/1 -> Divide10/2
  dynCoeff/1 -> Divide11/2
  p/1 -> Divide10/1
  Add2/1 -> Divide11/1
  Divide9/1 -> Add2/2
  Divide11/1 -> Yawing Moment/1
  r/1 -> Divide9/2
  Divide10/1 -> Add2/1
